simulink model "multi_direction_robot"  (R2023b)
settings: Solver=VariableStepAuto  StartTime=0.0  StopTime=10.0  RelTol=1e-3
undefined symbols (not defined in the file): d1, d2, initial_condition, R, w1, w2, w3, w4
settings Model: Creator=roman  LastModifiedBy=roman

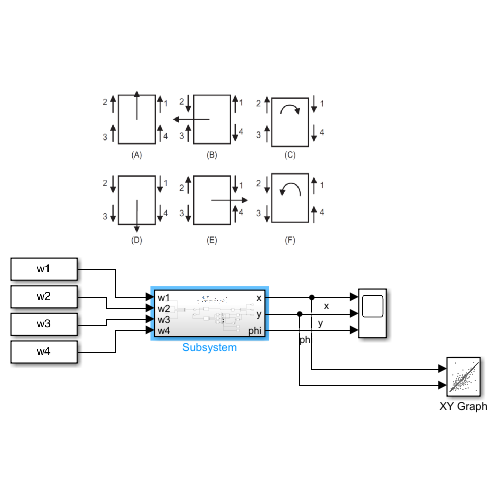
[thumbnail: Simulink's stored preview of the top-level diagram]
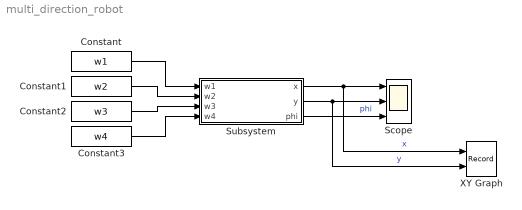
== system multi_direction_robot ==
  Constant : Constant  Value=w1
  Constant1 : Constant  Value=w2
  Constant2 : Constant  Value=w3
  Constant3 : Constant  Value=w4
  Scope : Scope  NumInputPorts=3
  Subsystem : Subsystem
  XY Graph : Record  FileSettingsInternal="{\"entries\":[{\"content\":{\"excelSettings\":{\"content\":{},\"type\":\"Streamout.ExcelSettings\"}},\"type\":\"Streamout.FileSettingStorage\",\"uuid\":\"\"}],\"packageUris\":[\"http:\\/\\/schema.mathworks.com\\/mf0\\/streamout_blocks\\/R2020a\"],\"version\":\"1.0\"}"  Layout=[1 1]  SignalsInternal="{\"entries\":[{\"content\":{\"signals\":[{\"content\":{\"blockPath\":[],\"dimensions\":[1],\"domain\":\"\",\"lineColor\":\"#a2142f\",\"plots\":[ 1 ],\"port\":1,\"sid\":[\"\"],\"signalID\":1,\"signalName\":\"x\"},\"type\":\"RecordBlkView.Signal\",\"uuid\":\"\"},{\"content\":{\"blockPath\":[],\"dimensions\":[1],\"domain\":\"\",\"lineColor\":\"#139fff\",\"plots\":[ 1 ],\"port\":2,\"sid\":[\"\"],\"signalID\":2,\"signalName\":\"y\"},\"type\":\"RecordBlkView.Signal\",\"uuid\":\"\"}]},\"type\":\"RecordBlkView.InputSignals\",\"uuid\":\"\"}],\"packageUris\":[\"http:\\/\\/schema.mathworks.com\\/mf0\\/streamout_blocks\\/R2020a\"],\"version\":\"1.0\"}"  VisualizationBindings="{\"xyplotplugin\":{\"info\":[{\"series\":[{\"bindingParametersList\":[{\"parameter\":\"X-Axis\",\"signalID\":1,\"signalName\":\"x\"},{\"parameter\":\"Y-Axis\",\"signalID\":2,\"signalName\":\"y\"}],\"seriesID\":0}],\"subplotID\":1}]}}"  CompatibilityTag=XY  st=-1
  wires:
  Subsystem/1(x) -> XY Graph/1, Scope/1  "x"
  Subsystem/2(y) -> XY Graph/2, Scope/2  "y"
  Subsystem/3(phi) -> Scope/3  "phi"
  Constant/1 -> Subsystem/1(w1)
  Constant1/1 -> Subsystem/2(w2)
  Constant2/1 -> Subsystem/3(w3)
  Constant3/1 -> Subsystem/4(w4)

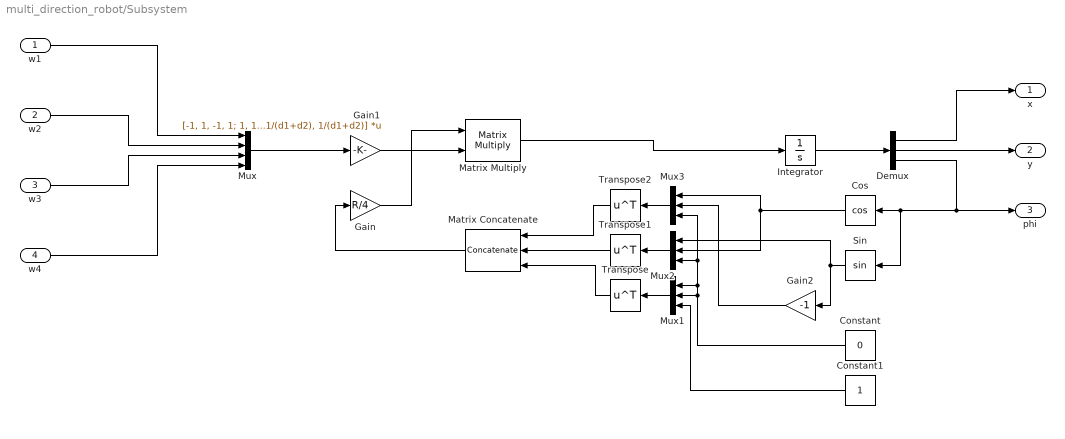
== system multi_direction_robot/Subsystem ==
  w1 : Inport
  w2 : Inport  Port=2
  w3 : Inport  Port=3
  w4 : Inport  Port=4
  Constant : Constant  Value=0
  Constant1 : Constant
  Cos : Trigonometry  Operator=cos  OutputSignalType=real
  Demux : Demux  Outputs=3
  Gain : Gain  Gain=R/4
  Gain1 : Gain  Gain=[-1, 1, -1, 1; 1, 1, 1, 1; 1/(d1+d2), -1/(d1+d2), -1/(d1+d2), 1/(d1+d2)]  Multiplication=Matrix(K*u)
  Gain2 : Gain  Gain=-1
  Integrator : Integrator  InitialCondition=initial_condition
  Matrix Concatenate : Concatenate  NumInputs=3  Mode=Multidimensional array
  Matrix Multiply : Product  Multiplication=Matrix(*)
  Mux : Mux
  Mux1 : Mux  Inputs=3
  Mux2 : Mux  Inputs=3
  Mux3 : Mux  Inputs=3
  Sin : Trigonometry  OutputSignalType=real
  Transpose : Math  Operator=transpose
  Transpose1 : Math  Operator=transpose
  Transpose2 : Math  Operator=transpose
  x : Outport
  y : Outport  Port=2
  phi : Outport  Port=3
  wires:
  Matrix Multiply/1 -> Integrator/1
  Integrator/1 -> Demux/1
  Demux/1 -> x/1
  Demux/2 -> y/1
  Demux/3 -> Cos/1, Sin/1, phi/1
  w1/1 -> Mux/1
  w2/1 -> Mux/2
  w3/1 -> Mux/3
  w4/1 -> Mux/4
  Mux/1 -> Gain1/1
  Sin/1 -> Mux2/1, Gain2/1
  Cos/1 -> Mux3/1, Mux2/2
  Gain2/1 -> Mux3/2
  Constant/1 -> Mux1/2, Mux1/1, Mux3/3, Mux2/3
  Matrix Concatenate/1 -> Gain/1
  Constant1/1 -> Mux1/3
  Gain/1 -> Matrix Multiply/1
  Gain1/1 -> Matrix Multiply/2
  Mux3/1 -> Transpose2/1
  Mux2/1 -> Transpose1/1
  Mux1/1 -> Transpose/1
  Transpose/1 -> Matrix Concatenate/3
  Transpose1/1 -> Matrix Concatenate/2
  Transpose2/1 -> Matrix Concatenate/1
